simulink model "Discrete_TF"  (R2017a)
settings: Solver=VariableStepAuto  StartTime=0.0  StopTime=500  RelTol=1e-3
values from neighbouring files (symbols this model uses):
  Ts = 0.21    [disc.m]    (also in inv_pend.m = 0.1)
settings Model: Creator=jdmor  LastModifiedBy=santiago

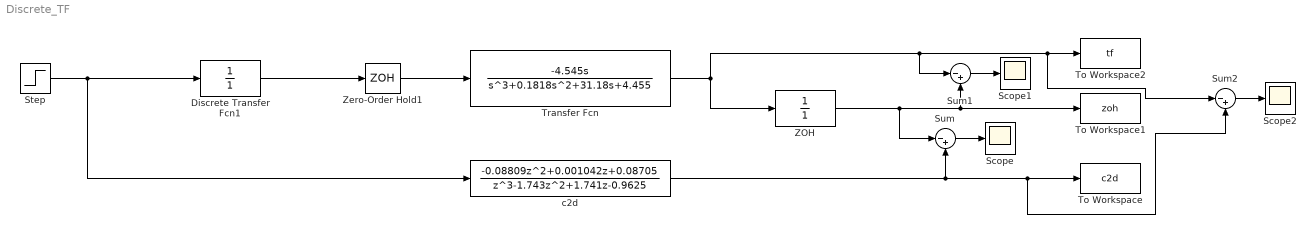
== system Discrete_TF ==
  Discrete Transfer Fcn1 : DiscreteTransferFcn  Denominator=[1]  SampleTime=Ts
  Scope : Scope
  Scope1 : Scope
  Scope2 : Scope
  Step : Step  SampleTime=0
  Sum : Sum  Inputs=|-+
  Sum1 : Sum  Inputs=|-+
  Sum2 : Sum  Inputs=|-+
  To Workspace : ToWorkspace  VariableName=c2d  SaveFormat=Timeseries  SampleTime=-1
  To Workspace1 : ToWorkspace  VariableName=zoh  SaveFormat=Timeseries  SampleTime=-1
  To Workspace2 : ToWorkspace  VariableName=tf  SaveFormat=Timeseries  SampleTime=-1
  Transfer Fcn : TransferFcn  Numerator=[-4.545 0]  Denominator=[1 0.1818 31.18 4.455]
  ZOH : DiscreteTransferFcn  Denominator=[1]  SampleTime=Ts
  Zero-Order Hold1 : ZeroOrderHold  SampleTime=Ts
  c2d : DiscreteTransferFcn  Numerator=[-0.08809 0.001042 0.08705]  Denominator=[1 -1.743 1.741 -0.9625]  SampleTime=Ts
  wires:
  Discrete Transfer Fcn1/1 -> Zero-Order Hold1/1
  Zero-Order Hold1/1 -> Transfer Fcn/1
  ZOH/1 -> Sum/1, Sum1/2, To Workspace1/1
  Step/1 -> c2d/1, Discrete Transfer Fcn1/1
  Sum/1 -> Scope/1
  Sum1/1 -> Scope1/1
  c2d/1 -> Sum/2, Sum2/2, To Workspace/1
  Sum2/1 -> Scope2/1
  Transfer Fcn/1 -> Sum1/1, Sum2/1, To Workspace2/1, ZOH/1
